simulink model "threephaserectifierusingdiodes"  (R2013a)
settings: Solver=ode45  StartTime=0.0  StopTime=.04  RelTol=1e-3
libraries: powerlib x16, powerlib_meascontrol x1, dspstat3 x1
settings Model: Creator=hp  LastModifiedBy=hp

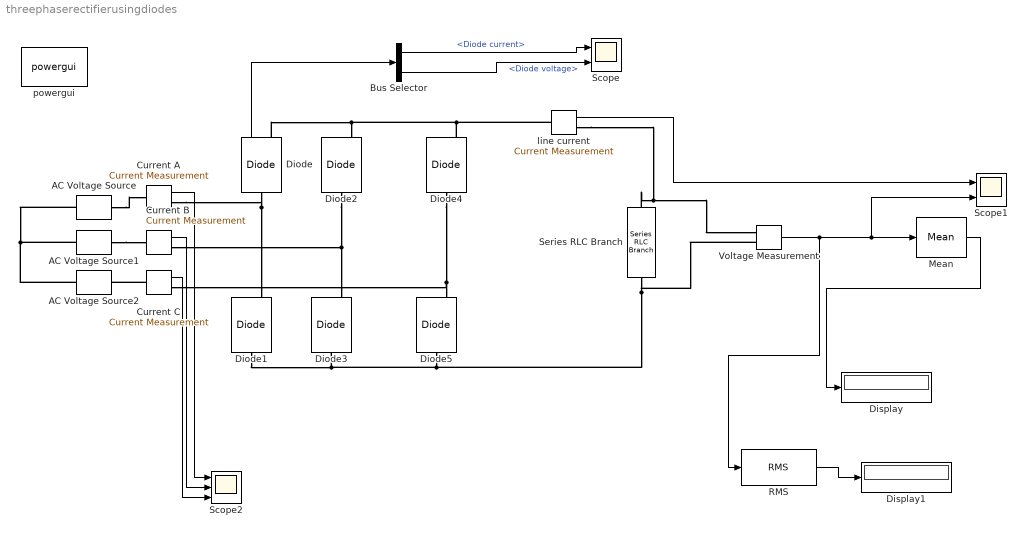
== system threephaserectifierusingdiodes ==
  AC Voltage Source : powerlib/Electrical Sources/AC Voltage Source  Amplitude=100  Phase=0  Frequency=50  SampleTime=0  Measurements=None
  AC Voltage Source1 : powerlib/Electrical Sources/AC Voltage Source  Amplitude=100  Phase=120  Frequency=50  SampleTime=0  Measurements=None
  AC Voltage Source2 : powerlib/Electrical Sources/AC Voltage Source  Amplitude=100  Phase=240  Frequency=50  SampleTime=0  Measurements=None
  Bus Selector : BusSelector  OutputSignals=Diode current,Diode voltage
  Current A : powerlib/Measurements/Current Measurement  PhasorSimulation=off  OutputType=Complex  PSBequivalent=0
  Current B : powerlib/Measurements/Current Measurement  PhasorSimulation=off  OutputType=Complex  PSBequivalent=0
  Current C : powerlib/Measurements/Current Measurement  PhasorSimulation=off  OutputType=Complex  PSBequivalent=0
  Diode{,1..5} (6 alike) : powerlib/Power Electronics/Diode  Ron=0.001  Lon=0  Vf=0.8  IC=0  UseSnubber=off  Rs=500  Cs=250e-9  Measurements=on
  Display : Display
      settings: Decimation=2
  Display1 : Display
      settings: Decimation=2
  Mean : powerlib_meascontrol/Measurements/Mean  Freq=60  Vinit=0  Ts=0
  RMS : dspstat3/RMS  run=off  reset_popup=None  InputProcessing=Columns as channels (frame based)  directionMode=Each column  dimension=1  treatSBRowAsCol=on
  Scope : Scope  NumInputPorts=2
      settings: YMin=-5~-5  YMax=5~5
  Scope1 : Scope  NumInputPorts=2
      settings: TimeRange=0.04  YMin=-5~-5  YMax=5~5  SaveName=voltage
  Scope2 : Scope  NumInputPorts=3
      settings: YMin=-5~-5~-5  YMax=5~5~5  SaveName=ScopeData2
  Series RLC Branch : powerlib/Elements/Series RLC Branch  LConnTagsString=__new0  RConnTagsString=__new0  BranchType=R  Resistance=10  Inductance=1e-3  SetiL0=off  InitialCurrent=0  Capacitance=1e-6  Setx0=off  InitialVoltage=0  Measurements=None
  Voltage Measurement : powerlib/Measurements/Voltage Measurement  PhasorSimulation=off  OutputType=Complex  PSBequivalent=0
  line current : powerlib/Measurements/Current Measurement  PhasorSimulation=off  OutputType=Complex  PSBequivalent=0
  powergui : powerlib/powergui  Priority=1  SimulationMode=Continuous  SolverType=Tustin  SampleTime=50e-6  frequency=60  SPID=off  DisableSnubberDevices=off  DisableRonSwitches=off  DisableVfSwitches=off  SwTol=0  Interpol=off  DisplayEquations=off  frequencyindice=50  Pbase=100e6  ErrMax=1e-4  Iterations=50  UnitsV=kV  UnitsW=MW  FunctionMessages=off  echomessages=off  HookPort=off  EnableUseOfTLC=off  x0status=blocks  RestoreLinks=warning  ResistiveCurrentMeasurement=off  Frange=[0:2:500]  Ylog=off  Xlog=on  ShowGrid=off  save=off  variable=ZData  structure=current  ZoomFFT=on  StartTime=0.0  cycles=1  DisplayStyle=2  fundamental=50  FreqAxis=off  MaxFrequency=1000  frequencyindicesteady=1  RmsSteady=1  display=off  Ts=0  methode=off
  wires:
  Voltage Measurement/1 -> RMS/1, Mean/1, Scope1/2
  line current/1 -> Scope1/1
  Diode/1 -> Bus Selector/1
  Bus Selector/1 -> Scope/1  "<Diode current>"
  Bus Selector/2 -> Scope/2  "<Diode voltage>"
  Current A/1 -> Scope2/1
  Current B/1 -> Scope2/2
  Current C/1 -> Scope2/3
  Mean/1 -> Display/1
  RMS/1 -> Display1/1
  connections:
  AC Voltage Source/LConn1 -- AC Voltage Source2/LConn1 -- AC Voltage Source1/LConn1
  Diode/LConn1 -- Diode1/RConn1 -- Current A/RConn1
  Diode2/LConn1 -- Current B/RConn1 -- Diode3/RConn1
  Diode4/LConn1 -- Current C/RConn1 -- Diode5/RConn1
  Series RLC Branch/RConn1 -- Diode5/LConn1 -- Diode1/LConn1 -- Diode3/LConn1 -- Voltage Measurement/LConn2
  Series RLC Branch/LConn1 -- line current/RConn1 -- Voltage Measurement/LConn1
  Diode4/RConn1 -- Diode/RConn1 -- Diode2/RConn1 -- line current/LConn1
  AC Voltage Source1/RConn1 -- Current B/LConn1
  AC Voltage Source/RConn1 -- Current A/LConn1
  Current C/LConn1 -- AC Voltage Source2/RConn1
